simulink model "q_qube2_swingup"  (R2021a)
settings: Solver=ode1  StartTime=0.0  StopTime=50  FixedStep=Ts  RelTol=1e-3  EnableMultiTasking=on
values from neighbouring files (symbols this model uses):
  layer1 = double(criticParams{1,1})    [setup_swingup.m]
  layer2 = double(criticParams{1,2})    [setup_swingup.m]
  layer3 = double(criticParams{1,3})    [setup_swingup.m]
  layer4 = double(criticParams{1,4})    [setup_swingup.m]
  layer5 = double(criticParams{1,5})    [setup_swingup.m]
  layer6 = double(criticParams{1,6})    [setup_swingup.m]
  nI = obsInfo.Dimension(1)    [setup_swingup.m]
  nL = 24    [setup_swingup.m]
  nO = 3    [setup_swingup.m]
  tau_max = kt*10/Rm    (= 0.05)    [qube2_rotpen_param.m]
undefined symbols (not defined in the file or in its folder): HIL, Q, qc_get_step_size, R
libraries: quarc_library x3
settings Model: SimulationMode=external  ExtModeTrigDuration=10000  Creator=MLevis
settings SolverCC: AlgebraicLoopSolver=TrustRegion  PositivePriorityOrder=on  AutoInsertRateTranBlk=on
settings DebuggingCC: UnderspecifiedInitializationDetection=Classic  MergeDetectMultiDrivingBlocksExec=none  SFMachineParentedDataDiag=warning
settings ModelReferenceCC: PropagateSignalLabelsOutOfModel=off
settings SFSimCC: CustomCodeUndefinedFunction=UseInterfaceOnly
settings RTWCC: Description=QUARC Win64 Target Using Toolchain  SystemTargetFile=quarc_win64.tlc  TemplateMakefile=quarc_default_tmf  Toolchain=QUARC win64 | nmake (64-bit Windows)  BuildConfiguration=Faster Runs
settings STFCustomTargetCC: TargetLangStandard=C99 (ISO)  ConcurrentExecutionCompliant=on  SystemTargetFile=quarc_win64.tlc
settings GRTTargetCC: ParMdlRefBuildCompliant=off  CompOptLevelCompliant=off  CombineOutputUpdateFcns=off  MatFileLogging=off  CPPClassGenCompliant=off  GRTInterface=on  ExtMode=on  ExtModeMexFile=quarc_comm

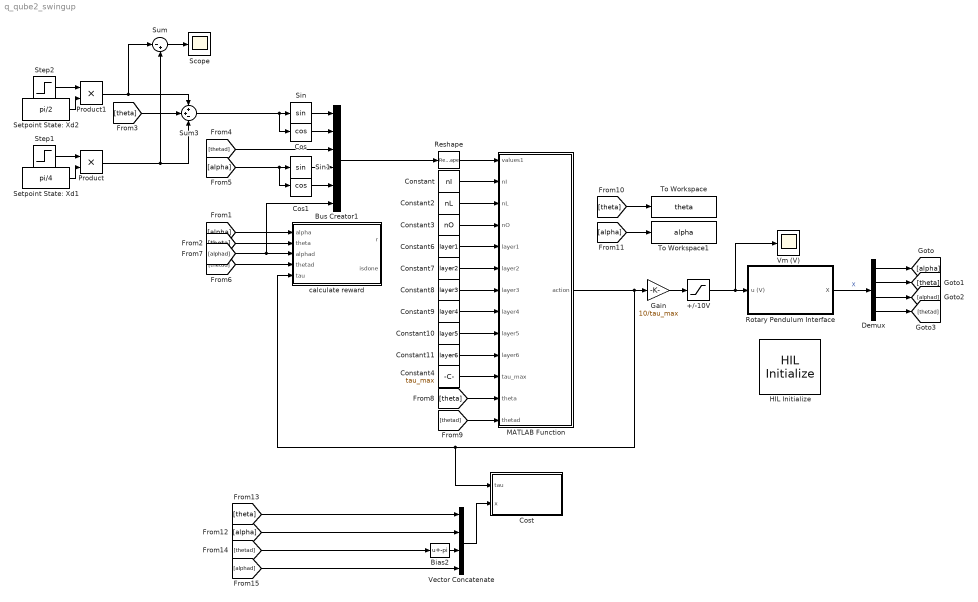
== system q_qube2_swingup ==
  +/-10V : Saturate  UpperLimit=10  LowerLimit=-10
  Bias2 : Bias  Bias=-pi
  Bus Creator1 : BusCreator  Inputs=6
  Constant : Constant  Value=nI
  Constant10 : Constant  Value=layer5
  Constant11 : Constant  Value=layer6
  Constant2 : Constant  Value=nL
  Constant3 : Constant  Value=nO
  Constant4 : Constant  Value=tau_max
  Constant6 : Constant  Value=layer1
  Constant7 : Constant  Value=layer2
  Constant8 : Constant  Value=layer3
  Constant9 : Constant  Value=layer4
  Cos : Trigonometry  Operator=cos
  Cos1 : Trigonometry  Operator=cos
  Cost : Subsystem
  Demux : Demux
  Gain : Gain  Gain=10/tau_max
  HIL Initialize : quarc_library/Data Acquisition/Generic/Configuration/HIL Initialize  object_name=HIL-1  board_type=qube_servo_usb  board_number=0  board_options=d0=pwm;d1=pwm;led=auto;update_rate=normal;decimation=1  exclusive=off  active=on  hardware_clocks=[0]  clock_modes=[]  initial_clock_frequencies=[]  set_clock_params_at_start=off  set_clock_params_at_switch_in=off  set_clock_frequencies_at_start=off  set_clock_frequencies_at_switch_in=off  analog_input_channels=[]  analog_input_configurations=[]  analog_input_maximums=[]  analog_input_minimums=[]  set_analog_input_params_at_start=off  set_analog_input_params_at_switch_in=off  analog_output_channels=0  analog_output_maximums=10  analog_output_minimums=-10  initial_analog_outputs=[0]  final_analog_outputs=[0]  watchdog_analog_outputs=0  set_analog_output_params_at_start=on  set_analog_output_params_at_switch_in=off  set_analog_outputs_at_start=on  set_analog_outputs_at_switch_in=off  set_analog_outputs_at_terminate=on  set_analog_outputs_at_switch_out=off  set_analog_outputs_on_watchdog=off  digital_input_channels=[]  digital_output_channels=[]  digital_output_configuration=[]  initial_digital_outputs=[]  final_digital_outputs=[]  watchdog_digital_outputs=[]  set_digital_output_params_at_start=off  set_digital_output_params_at_switch_in=off  set_digital_outputs_at_start=off  set_digital_outputs_at_switch_in=off  set_digital_outputs_at_terminate=off  set_digital_outputs_at_switch_out=off  set_digital_outputs_on_watchdog=off  encoder_channels=[0:1]  quadrature=[4]  encoder_filter_frequency=[]  initial_encoder_counts=[0]  set_encoder_params_at_start=on  set_encoder_params_at_switch_in=off  set_encoder_counts_at_start=on  set_encoder_counts_at_switch_in=off  pwm_channels=[]  pwm_modes=[]  pwm_frequency=[]  pwm_configuration=[]  pwm_alignment=[]  pwm_polarity=[]  pwm_leading_deadband=[]  pwm_trailing_deadband=[]  initial_pwm_outputs=[]  final_pwm_outputs=[]  watchdog_pwm_outputs=[]  set_pwm_params_at_start=off  set_pwm_params_at_switch_in=off  set_pwm_outputs_at_start=off  set_pwm_outputs_at_switch_in=off  set_pwm_outputs_at_terminate=off  set_pwm_outputs_at_switch_out=off  set_pwm_outputs_on_watchdog=off  other_output_channels=[]  initial_other_outputs=[]  final_other_outputs=[]  watchdog_other_outputs=[]  set_other_outputs_at_start=off  set_other_outputs_at_switch_in=off  set_other_outputs_at_terminate=off  set_other_outputs_at_switch_out=off  set_other_outputs_on_watchdog=off
  MATLAB Function : MATLAB Function  TreatAsAtomicUnit=on
  Product : Product
  Product1 : Product
  Reshape : Reshape  OutputDimensionality=Row vector (2-D)
  Rotary Pendulum Interface : Subsystem
  Scope : Scope
  Setpoint State: Xd1 : Constant  Value=pi/4
  Setpoint State: Xd2 : Constant  Value=pi/2
  Sin : Trigonometry
  Sin1 : Trigonometry
  Step1 : Step  Time=10  SampleTime=0
  Step2 : Step  Time=20  SampleTime=0
  Sum : Sum  Inputs=|-+
  Sum3 : Sum  Inputs=++-
  To Workspace : ToWorkspace  VariableName=theta  SaveFormat=Timeseries  SampleTime=-1
  To Workspace1 : ToWorkspace  VariableName=alpha  SaveFormat=Timeseries  SampleTime=-1
  Vector Concatenate : Concatenate  NumInputs=4
  Vm (V) : Scope
  calculate reward : Subsystem
  wires:
  Rotary Pendulum Interface/1(X) -> Demux/1  "X"
  Gain/1 -> +/-10V/1
  Demux/1 -> [alpha]
  Demux/3 -> [alphad]
  Demux/4 -> [thetad]
  [theta] -> To Workspace/1
  +/-10V/1 -> Vm (V)/1, Rotary Pendulum Interface/1(u (V))
  [alpha] -> To Workspace1/1
  [alphad] -> Bus Creator1/6, calculate reward/3(alphad)
  [thetad] -> calculate reward/4(thetad)
  [theta] -> calculate reward/2(theta)
  [alpha] -> calculate reward/1(alpha)
  [alpha] -> Cos1/1, Sin1/1
  [thetad] -> Bus Creator1/3
  Sin1/1 -> Bus Creator1/4
  Sin/1 -> Bus Creator1/1
  Cos/1 -> Bus Creator1/2
  Cos1/1 -> Bus Creator1/5
  Constant4/1 -> MATLAB Function/11(tau_max)
  Constant3/1 -> MATLAB Function/4(nO)
  Constant6/1 -> MATLAB Function/5(layer1)
  Constant7/1 -> MATLAB Function/6(layer2)
  Constant2/1 -> MATLAB Function/3(nL)
  Constant8/1 -> MATLAB Function/7(layer3)
  Constant10/1 -> MATLAB Function/9(layer5)
  Bus Creator1/1 -> Reshape/1
  Constant9/1 -> MATLAB Function/8(layer4)
  Constant/1 -> MATLAB Function/2(nI)
  Constant11/1 -> MATLAB Function/10(layer6)
  Reshape/1 -> MATLAB Function/1(values1)
  [theta] -> MATLAB Function/12(theta)
  [thetad] -> MATLAB Function/13(thetad)
  [alpha] -> Vector Concatenate/2
  [alphad] -> Vector Concatenate/4
  Bias2/1 -> Vector Concatenate/3
  Vector Concatenate/1 -> Cost/2(x)
  [thetad] -> Bias2/1
  [theta] -> Vector Concatenate/1
  MATLAB Function/1(action) -> Cost/1(tau), calculate reward/5(tau), Gain/1
  Demux/2 -> [theta]
  Sum/1 -> Scope/1
  Sum3/1 -> Cos/1, Sin/1
  Product1/1 -> Sum/1, Sum3/1
  Step1/1 -> Product/1
  Setpoint State: Xd1/1 -> Product/2
  Step2/1 -> Product1/1
  Product/1 -> Sum/2, Sum3/3
  Setpoint State: Xd2/1 -> Product1/2
  [theta] -> Sum3/2

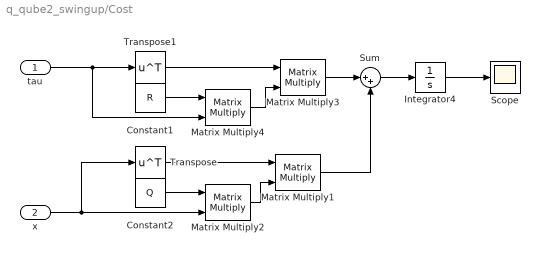
== system q_qube2_swingup/Cost ==
  tau : Inport
  x : Inport  Port=2
  Constant1 : Constant  Value=R
  Constant2 : Constant  Value=Q
  Integrator4 : Integrator
  Matrix Multiply{1..4} (4 alike) : Product  Multiplication=Matrix(*)
  Scope : Scope
  Sum : Sum  Inputs=|++
  Transpose : Math  Operator=transpose  SaturateOnIntegerOverflow=on
  Transpose1 : Math  Operator=transpose  SaturateOnIntegerOverflow=on
  wires:
  Transpose/1 -> Matrix Multiply1/1
  Matrix Multiply2/1 -> Matrix Multiply1/2
  Integrator4/1 -> Scope/1
  x/1 -> Matrix Multiply2/2, Transpose/1
  Constant2/1 -> Matrix Multiply2/1
  Matrix Multiply1/1 -> Sum/2
  Sum/1 -> Integrator4/1
  Matrix Multiply3/1 -> Sum/1
  Constant1/1 -> Matrix Multiply4/1
  Transpose1/1 -> Matrix Multiply3/1
  Matrix Multiply4/1 -> Matrix Multiply3/2
  tau/1 -> Matrix Multiply4/2, Transpose1/1

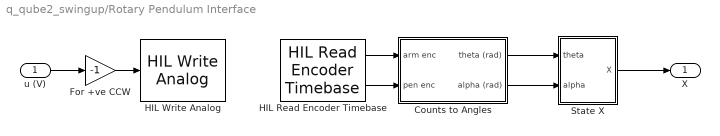
== system q_qube2_swingup/Rotary Pendulum Interface ==
  u (V) : Inport
  Counts to Angles : Subsystem
  For +ve CCW : Gain  Gain=-1
  HIL Read Encoder Timebase : quarc_library/Data Acquisition/Generic/Timebases/HIL Read Encoder Timebase  object_name=HIL-1  clock=0  channels=[0:1]  active=on  vector_output=off  data_type_mode=Inherit via back propagation  data_type=double  overflow_mode=Error on overflow  samples_in_buffer=max(ceil(1/qc_get_step_size), 1)
  HIL Write Analog : quarc_library/Data Acquisition/Generic/Immediate I//O/HIL Write Analog  object_name=HIL-1  channels=0  sample_time=-1  active=on  vector_input=off
  State X : Subsystem
  X : Outport  VectorParamsAs1DForOutWhenUnconnected=off
  wires:
  For +ve CCW/1 -> HIL Write Analog/1
  Counts to Angles/2(alpha (rad)) -> State X/2(alpha)
  Counts to Angles/1(theta (rad)) -> State X/1(theta)
  State X/1(X) -> X/1
  u (V)/1 -> For +ve CCW/1
  HIL Read Encoder Timebase/1 -> Counts to Angles/1(arm enc)
  HIL Read Encoder Timebase/2 -> Counts to Angles/2(pen enc)

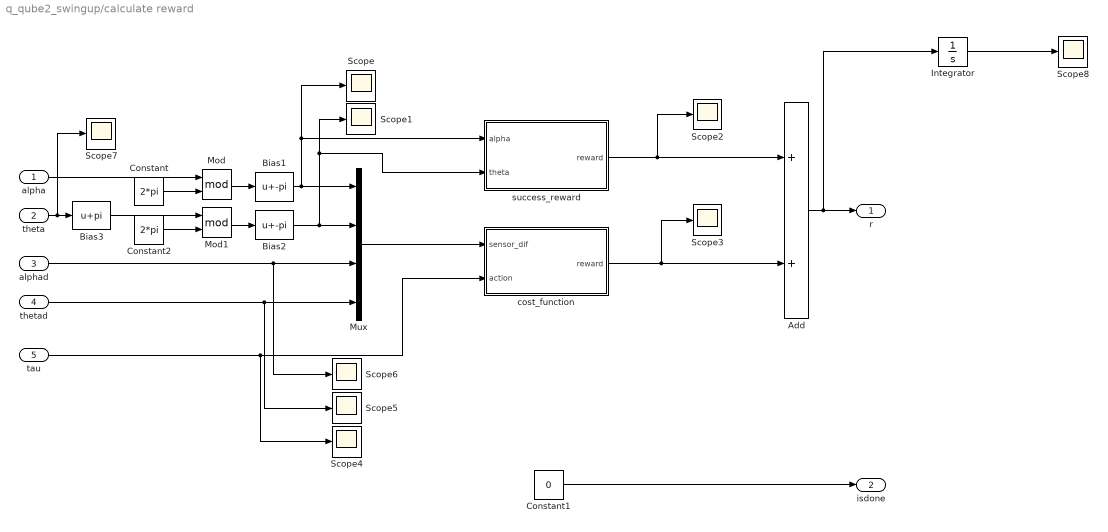
== system q_qube2_swingup/calculate reward ==
  alpha : Inport
  theta : Inport  Port=2
  alphad : Inport  Port=3
  thetad : Inport  Port=4
  tau : Inport  Port=5
  Add : Sum
  Bias1 : Bias  Bias=-pi
  Bias2 : Bias  Bias=-pi
  Bias3 : Bias  Bias=pi
  Constant : Constant  Value=2*pi
  Constant1 : Constant  Value=0
  Constant2 : Constant  Value=2*pi
  Integrator : Integrator
  Mod : Math  Operator=mod  SaturateOnIntegerOverflow=on
  Mod1 : Math  Operator=mod  SaturateOnIntegerOverflow=on
  Mux : Mux
  Scope{,1..8} (9 alike) : Scope
  cost_function : Subsystem
  success_reward : Subsystem
  r : Outport  VectorParamsAs1DForOutWhenUnconnected=off
  isdone : Outport  Port=2  VectorParamsAs1DForOutWhenUnconnected=off
  wires:
  Constant/1 -> Mod/2
  Mod/1 -> Bias1/1
  alpha/1 -> Mod/1
  Bias1/1 -> success_reward/1(alpha), Scope/1, Mux/1
  alphad/1 -> Scope6/1, Mux/3
  tau/1 -> Scope4/1, cost_function/2(action)
  Mux/1 -> cost_function/1(sensor_dif)
  success_reward/1(reward) -> Scope2/1, Add/1
  cost_function/1(reward) -> Scope3/1, Add/2
  Constant1/1 -> isdone/1
  Constant2/1 -> Mod1/2
  theta/1 -> Scope7/1, Bias3/1
  Mod1/1 -> Bias2/1
  Bias2/1 -> Scope1/1, success_reward/2(theta), Mux/2
  Bias3/1 -> Mod1/1
  thetad/1 -> Scope5/1, Mux/4
  Add/1 -> Integrator/1, r/1
  Integrator/1 -> Scope8/1

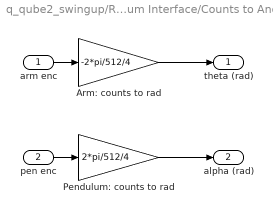
== system q_qube2_swingup/Rotary Pendulum Interface/Counts to Angles ==
  arm enc : Inport
  pen enc : Inport  Port=2
  Arm: counts to rad : Gain  Gain=-2*pi/512/4
  Pendulum: counts to rad : Gain  Gain=2*pi/512/4
  theta (rad) : Outport  VectorParamsAs1DForOutWhenUnconnected=off
  alpha (rad) : Outport  Port=2  VectorParamsAs1DForOutWhenUnconnected=off
  wires:
  pen enc/1 -> Pendulum: counts to rad/1
  arm enc/1 -> Arm: counts to rad/1
  Arm: counts to rad/1 -> theta (rad)/1
  Pendulum: counts to rad/1 -> alpha (rad)/1

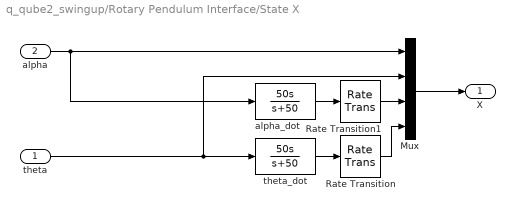
== system q_qube2_swingup/Rotary Pendulum Interface/State X ==
  theta : Inport
  alpha : Inport  Port=2
  Mux : Mux
  Rate Transition : RateTransition
  Rate Transition1 : RateTransition
  alpha_dot : TransferFcn  Numerator=[50 0]  Denominator=[1 50]
  theta_dot : TransferFcn  Numerator=[50 0]  Denominator=[1 50]
  X : Outport  VectorParamsAs1DForOutWhenUnconnected=off
  wires:
  Mux/1 -> X/1
  theta/1 -> Mux/2, theta_dot/1
  alpha/1 -> Mux/1, alpha_dot/1
  theta_dot/1 -> Rate Transition/1
  Rate Transition/1 -> Mux/4
  alpha_dot/1 -> Rate Transition1/1
  Rate Transition1/1 -> Mux/3

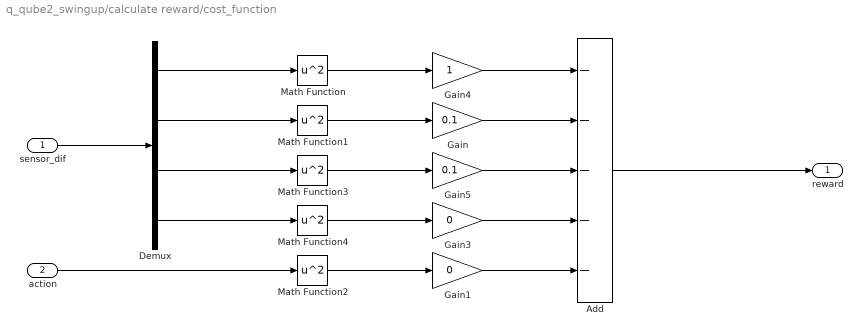
== system q_qube2_swingup/calculate reward/cost_function ==
  sensor_dif : Inport
  action : Inport  Port=2
  Add : Sum  Inputs=-----
  Demux : Demux
  Gain : Gain  Gain=0.1
  Gain1 : Gain  Gain=0
  Gain3 : Gain  Gain=0
  Gain4 : Gain
  Gain5 : Gain  Gain=0.1
  Math Function{,1..4} (5 alike) : Math  Operator=square  SaturateOnIntegerOverflow=on
  reward : Outport
  wires:
  Math Function4/1 -> Gain3/1
  Gain3/1 -> Add/4
  Gain1/1 -> Add/5
  Add/1 -> reward/1
  sensor_dif/1 -> Demux/1
  Demux/4 -> Math Function4/1
  Demux/3 -> Math Function3/1
  Demux/2 -> Math Function1/1
  Math Function1/1 -> Gain/1
  Math Function3/1 -> Gain5/1
  action/1 -> Math Function2/1
  Demux/1 -> Math Function/1
  Math Function2/1 -> Gain1/1
  Gain4/1 -> Add/1
  Gain5/1 -> Add/3
  Gain/1 -> Add/2
  Math Function/1 -> Gain4/1

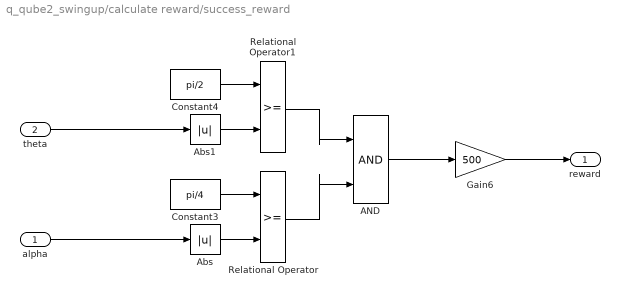
== system q_qube2_swingup/calculate reward/success_reward ==
  alpha : Inport
  theta : Inport  Port=2
  AND : Logic  IconShape=distinctive  AllPortsSameDT=off  OutDataTypeStr=boolean
  Abs : Abs
  Abs1 : Abs
  Constant3 : Constant  Value=pi/4
  Constant4 : Constant  Value=pi/2
  Gain6 : Gain  Gain=500
  Relational Operator : RelationalOperator  OutDataTypeStr=boolean  RndMeth=Simplest
  Relational Operator1 : RelationalOperator  OutDataTypeStr=boolean  RndMeth=Simplest
  reward : Outport
  wires:
  Gain6/1 -> reward/1
  Constant3/1 -> Relational Operator/1
  Abs/1 -> Relational Operator/2
  AND/1 -> Gain6/1
  Relational Operator/1 -> AND/2
  Abs1/1 -> Relational Operator1/2
  Constant4/1 -> Relational Operator1/1
  Relational Operator1/1 -> AND/1
  alpha/1 -> Abs/1
  theta/1 -> Abs1/1

== matlab function q_qube2_swingup/MATLAB Function ==
  data: values1 input; action output; nI input; nL input; nO input; layer1 input; layer2 input; layer3 input; layer4 input; layer5 input; layer6 input; tau_max input; theta input; thetad input
function action = fcn(values1,nI,nL,nO,layer1,layer2,layer3,layer4,layer5,layer6,tau_max,theta,thetad)

values2 = zeros(1,size(layer1,1));
for j = 1:size(layer1,1)
    values2(1,j) = fullyConnected(layer1(j,:),values1,layer2(j));
end

values3 = ReLu(values2);

values4 = zeros(1,size(layer3,1));
for j = 1:size(layer3,1)
    values4(1,j) = fullyConnected(layer3(j,:),values3,layer4(j));
end

values5 = ReLu(values4);

values6 = zeros(1,size(layer5,1));
for j = 1:size(layer5,1)
    values6(1,j) = fullyConnected(layer5(j,:),values5,layer6(j));
end
values7 = ReLu(values6);

[maxValue, maxIndex] = max(values6);
action = (maxIndex-2) * tau_max;

if theta > 0.65*pi && thetad > -5
    action = -tau_max;
elseif theta < -0.65*pi && thetad < 5
    action = tau_max;
end

end
